simulink model "pfc_closed_loop_ripple4"  (R2016b)
settings: Solver=VariableStepAuto  StartTime=0.0  StopTime=1  RelTol=1e-3
libraries: powerlib x27, simulink x5, powerlib_meascontrol x4
settings Model: SimulationMode=accelerator  Creator=exam  LastModifiedBy=Saagar
settings SolverCC: ZeroCrossAlgorithm=Adaptive

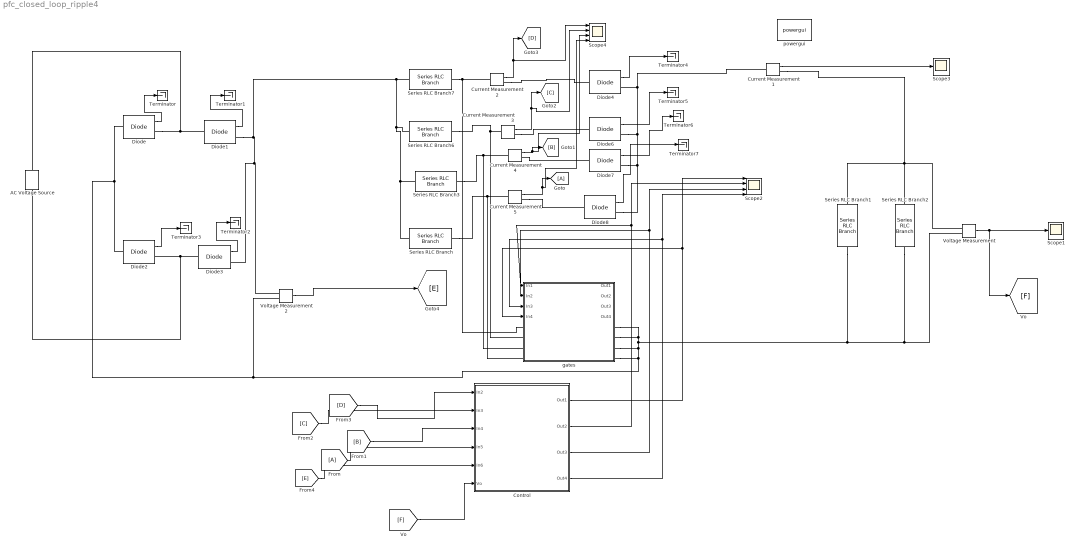
== system pfc_closed_loop_ripple4 ==
  AC Voltage Source : powerlib/Electrical Sources/AC Voltage Source  Amplitude=325  Phase=0  Frequency=50  SampleTime=0  Measurements=None  BusType=swing  Pref=10e3  Qref=0  Qmin=-inf  Qmax=+inf
  Control : Subsystem
  Current Measurement{1..5} (5 alike) : powerlib/Measurements/Current Measurement  PhasorSimulation=off  OutputType=Complex  PSBequivalent=0
  Diode{,1,3..4,6..8} (7 alike) : powerlib/Power Electronics/Diode  Ron=0.001  Lon=0  Vf=0.8  IC=0  UseSnubber=off  Rs=500  Cs=250e-9  Measurements=on
  Diode2 : powerlib/Power Electronics/Diode  Ron=0.001  Lon=0  Vf=0.6  IC=0  UseSnubber=off  Rs=500  Cs=250e-9  Measurements=on
  Scope1 : Scope
  Scope2 : Scope  NumInputPorts=4
  Scope3 : Scope
  Scope4 : Scope  NumInputPorts=4
  Series RLC Branch{,3,6..7} (4 alike) : powerlib/Elements/Series RLC Branch  LConnTagsString=__new0  RConnTagsString=__new0  BranchType=L  Resistance=0  Inductance=0.152e-03  SetiL0=off  InitialCurrent=0  Capacitance=0  Setx0=off  InitialVoltage=0  Measurements=None
  Series RLC Branch1 : powerlib/Elements/Series RLC Branch  LConnTagsString=__new0  RConnTagsString=__new0  BranchType=C  Resistance=0  Inductance=0  SetiL0=off  InitialCurrent=0  Capacitance=4700e-06  Setx0=off  InitialVoltage=0  Measurements=None
  Series RLC Branch2 : powerlib/Elements/Series RLC Branch  LConnTagsString=__new0  RConnTagsString=__new0  BranchType=R  Resistance=150  Inductance=0  SetiL0=off  InitialCurrent=0  Capacitance=10  Setx0=off  InitialVoltage=0  Measurements=None
  Terminator{,1..7} (8 alike) : Terminator
  Voltage Measurement : powerlib/Measurements/Voltage Measurement  PhasorSimulation=off  OutputType=Complex  PSBequivalent=0
  Voltage Measurement2 : powerlib/Measurements/Voltage Measurement  PhasorSimulation=off  OutputType=Complex  PSBequivalent=0
  gates : Subsystem
  powergui : powerlib/powergui  Priority=1  SimulationMode=Continuous  SolverType=Tustin/Backward Euler (TBE)  SampleTime=50e-6  frequency=60  SPID=off  DisableSnubberDevices=off  DisableRonSwitches=off  DisableVfSwitches=off  SwTol=0  DisplayEquations=off  Interpol=off  ExternalGateDelay=off  methode=off  Ts=10  FunctionMessages=off  echomessages=off  HookPort=off  EnableUseOfTLC=off  x0status=blocks  frequencyindice=0  Pbase=100e6  ErrMax=1e-4  Iterations=50  UnitsV=kV  UnitsW=MW  buscounter=0  RestoreLinks=warning  ResistiveCurrentMeasurement=off  Frange=[0:2:500]  Ylog=off  Xlog=on  ShowGrid=off  save=off  variable=ZData  structure=0  ZoomFFT=off  StartTime=0.0  cycles=1  DisplayStyle=1  fundamental=60  FreqAxis=off  MaxFrequency=1000  frequencyindicesteady=1  RmsSteady=1  display=off
  wires:
  Current Measurement1/1 -> Scope3/1
  Voltage Measurement/1 -> Scope1/1, [F]
  Current Measurement2/1 -> Scope4/1, [D]
  Current Measurement5/1 -> Scope4/4, [A]
  Current Measurement4/1 -> Scope4/3, [B]
  Current Measurement3/1 -> Scope4/2, [C]
  Control/4(Out4) -> Scope2/4, gates/3(In3)
  Control/1(Out1) -> Scope2/1, gates/4(In4)
  Control/2(Out2) -> gates/1(In1), Scope2/2
  Control/3(Out3) -> gates/2(In2), Scope2/3
  [D] -> Control/1(In2)
  [C] -> Control/2(In3)
  [B] -> Control/3(In4)
  [A] -> Control/4(In5)
  [E] -> Control/5(In6)
  [F] -> Control/6(Vo)
  Diode/1 -> Terminator/1
  Diode1/1 -> Terminator1/1
  Diode2/1 -> Terminator3/1
  Diode3/1 -> Terminator2/1
  Diode4/1 -> Terminator4/1
  Diode6/1 -> Terminator5/1
  Diode7/1 -> Terminator6/1
  Diode8/1 -> Terminator7/1
  Voltage Measurement2/1 -> [E]
  connections:
  Voltage Measurement/LConn1 -- Series RLC Branch1/LConn1 -- Current Measurement1/RConn1 -- Series RLC Branch2/LConn1
  Diode/RConn1 -- AC Voltage Source/RConn1 -- Diode1/LConn1
  Diode2/RConn1 -- AC Voltage Source/LConn1 -- Diode3/LConn1
  Voltage Measurement/LConn2 -- Series RLC Branch2/RConn1 -- Series RLC Branch1/RConn1 -- Diode2/LConn1 -- Diode/LConn1 -- Voltage Measurement2/LConn2 -- gates/RConn4 -- gates/RConn3 -- gates/RConn1 -- gates/RConn2
  Series RLC Branch7/RConn1 -- gates/LConn1 -- Current Measurement2/LConn1
  Diode7/RConn1 -- Current Measurement1/LConn1 -- Diode4/RConn1 -- Diode6/RConn1 -- Diode8/RConn1
  Current Measurement3/RConn1 -- Diode6/LConn1
  Current Measurement4/RConn1 -- Diode7/LConn1
  Current Measurement5/RConn1 -- Diode8/LConn1
  Series RLC Branch6/RConn1 -- Current Measurement3/LConn1 -- gates/LConn2
  Current Measurement5/LConn1 -- Series RLC Branch/RConn1 -- gates/LConn4
  Series RLC Branch3/RConn1 -- Current Measurement4/LConn1 -- gates/LConn3
  Current Measurement2/RConn1 -- Diode4/LConn1
  Diode1/RConn1 -- Series RLC Branch6/LConn1 -- Series RLC Branch/LConn1 -- Series RLC Branch3/LConn1 -- Series RLC Branch7/LConn1 -- Diode3/RConn1 -- Voltage Measurement2/LConn1

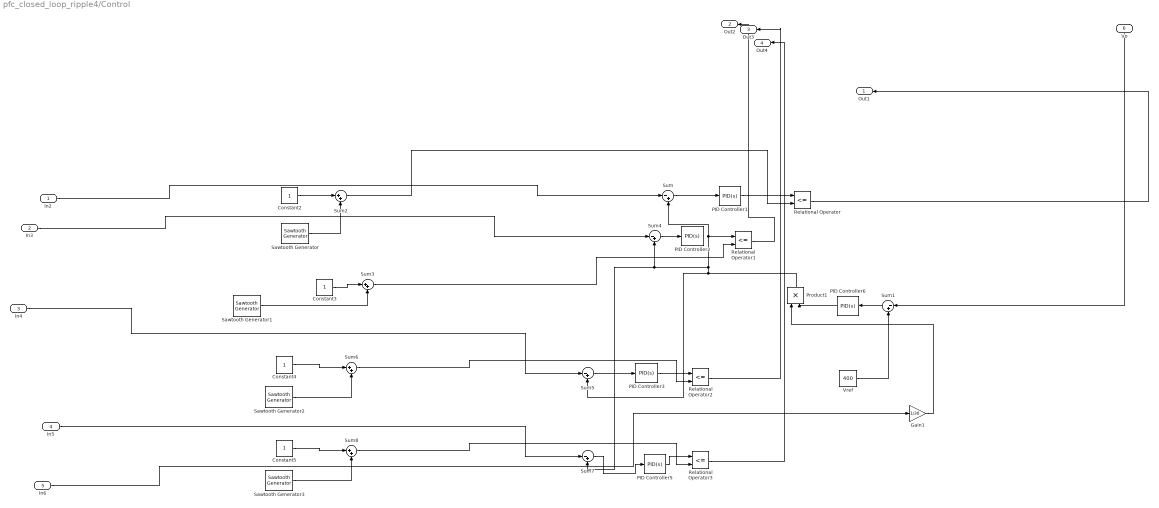
== system pfc_closed_loop_ripple4/Control ==
  In2 : Inport
  In3 : Inport  Port=2
  In4 : Inport  Port=3
  In5 : Inport  Port=4
  In6 : Inport  Port=5
  Vo : Inport  Port=6
  Constant{2..5} (4 alike) : Constant
  Gain1 : Gain  Gain=1/30
  PID Controller{1..3,5..6} (5 alike) : simulink/Continuous/PID Controller  Controller=PID  TimeDomain=Continuous-time  SampleTime=-1  IntegratorMethod=Forward Euler  FilterMethod=Forward Euler  Form=Parallel  UseFilter=on  ControllerParametersSource=internal  P=10  I=10  D=2.5  N=100  InitialConditionSource=internal  InitialConditionForIntegrator=0  InitialConditionForFilter=0  ExternalReset=none  LimitOutput=off  UpperSaturationLimit=inf  LowerSaturationLimit=-inf  LinearizeAsGain=on  AntiWindupMode=none  Kb=1  TrackingMode=off  Kt=1  PParamMin=[]  PParamMax=[]  IParamMin=[]  IParamMax=[]  DParamMin=[]  DParamMax=[]  NParamMin=[]  NParamMax=[]  KbParamMin=[]  KbParamMax=[]  KtParamMin=[]  KtParamMax=[]  POutMin=[]  POutMax=[]  IOutMin=[]  IOutMax=[]  DOutMin=[]  DOutMax=[]  NOutMin=[]  NOutMax=[]  KbOutMin=[]  KbOutMax=[]  KtOutMin=[]  KtOutMax=[]  IntegratorOutMin=[]  IntegratorOutMax=[]  FilterOutMin=[]  FilterOutMax=[]  SumOutMin=[]  SumOutMax=[]  SumI1OutMin=[]  SumI1OutMax=[]  SumI2OutMin=[]  SumI2OutMax=[]  SumI3OutMin=[]  SumI3OutMax=[]  SumDOutMin=[]  SumDOutMax=[]  SaturationOutMin=[]  SaturationOutMax=[]  IntegratorContinuousStateAttributes=''  IntegratorStateMustResolveToSignalObject=off  IntegratorRTWStateStorageClass=Auto  FilterContinuousStateAttributes=''  FilterStateMustResolveToSignalObject=off  FilterRTWStateStorageClass=Auto  DifferentiatorICPrevScaledInput=0  DifferentiatorOutMin=[]  DifferentiatorOutMax=[]
  Product1 : Product
  Relational Operator{,1..3} (4 alike) : RelationalOperator  Operator=<=  OutDataTypeStr=boolean  RndMeth=Simplest
  Sawtooth Generator : powerlib_meascontrol/Pulse & Signal Generators/Sawtooth Generator  Freq=40000  Phase=0  Ts=0
  Sawtooth Generator1 : powerlib_meascontrol/Pulse & Signal Generators/Sawtooth Generator  Freq=40000  Phase=90  Ts=0
  Sawtooth Generator2 : powerlib_meascontrol/Pulse & Signal Generators/Sawtooth Generator  Freq=40000  Phase=180  Ts=0
  Sawtooth Generator3 : powerlib_meascontrol/Pulse & Signal Generators/Sawtooth Generator  Freq=40000  Phase=270  Ts=0
  Sum{,1,4..5,7} (5 alike) : Sum  Inputs=|-+
  Sum{2..3,6,8} (4 alike) : Sum  Inputs=|++
  Vref : Constant  Value=400
  Out1 : Outport
  Out2 : Outport  Port=2
  Out3 : Outport  Port=3
  Out4 : Outport  Port=4
  wires:
  PID Controller6/1 -> Product1/2
  Sum/1 -> PID Controller1/1
  Sawtooth Generator/1 -> Sum2/2
  Constant3/1 -> Sum3/1
  Sawtooth Generator1/1 -> Sum3/2
  Sum3/1 -> Relational Operator1/2
  Constant2/1 -> Sum2/1
  Gain1/1 -> Product1/1
  Sum2/1 -> Relational Operator/2
  PID Controller1/1 -> Relational Operator/1
  Relational Operator/1 -> Out1/1
  Sum1/1 -> PID Controller6/1
  Sum5/1 -> PID Controller3/1
  Relational Operator3/1 -> Out4/1
  Sum8/1 -> Relational Operator3/2
  Relational Operator1/1 -> Out2/1
  Constant5/1 -> Sum8/1
  PID Controller5/1 -> Relational Operator3/1
  Relational Operator2/1 -> Out3/1
  Sum4/1 -> PID Controller2/1
  Sawtooth Generator2/1 -> Sum6/2
  Sum6/1 -> Relational Operator2/2
  PID Controller3/1 -> Relational Operator2/1
  Constant4/1 -> Sum6/1
  Product1/1 -> Sum5/2, Sum7/2, Sum4/2, Relational Operator1/1, Sum/2
  Sum7/1 -> PID Controller5/1
  Sawtooth Generator3/1 -> Sum8/2
  Vo/1 -> Sum1/1
  In5/1 -> Sum7/1
  In6/1 -> Gain1/1
  In2/1 -> Sum/1
  In4/1 -> Sum5/1
  In3/1 -> Sum4/1
  Vref/1 -> Sum1/2

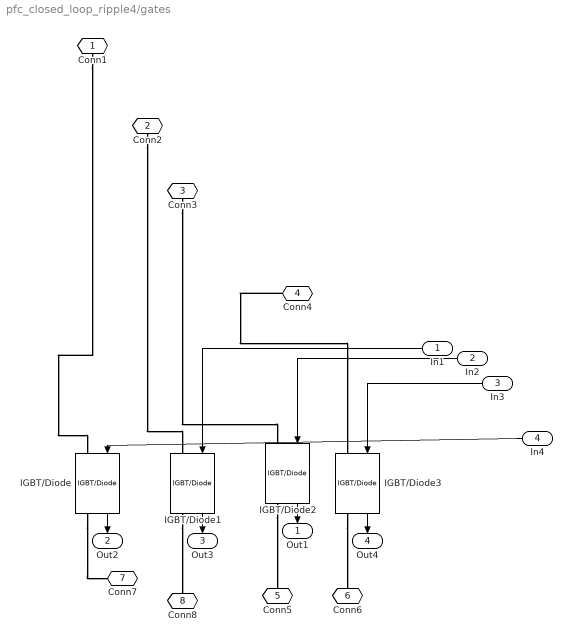
== system pfc_closed_loop_ripple4/gates ==
  In1 : Inport
  In2 : Inport  Port=2
  In3 : Inport  Port=3
  In4 : Inport  Port=4
  IGBT/Diode{,1..3} (4 alike) : powerlib/Power Electronics/IGBT//Diode  Ron=1e-3  Rs=1e5  Cs=inf  Measurements=on
  Conn1 : PMIOPort  Port=1  Side=Left
  Conn2 : PMIOPort  Port=2  Side=Left
  Conn3 : PMIOPort  Port=3  Side=Left
  Conn4 : PMIOPort  Port=4  Side=Left
  Conn5 : PMIOPort  Port=5  Side=Right
  Conn6 : PMIOPort  Port=6  Side=Right
  Conn7 : PMIOPort  Port=7  Side=Right
  Conn8 : PMIOPort  Port=8  Side=Right
  Out1 : Outport
  Out2 : Outport  Port=2
  Out3 : Outport  Port=3
  Out4 : Outport  Port=4
  wires:
  IGBT/Diode/1 -> Out2/1
  IGBT/Diode1/1 -> Out3/1
  IGBT/Diode2/1 -> Out1/1
  In3/1 -> IGBT/Diode3/1
  In1/1 -> IGBT/Diode1/1
  In2/1 -> IGBT/Diode2/1
  IGBT/Diode3/1 -> Out4/1
  In4/1 -> IGBT/Diode/1
  connections:
  IGBT/Diode3/RConn1 -- Conn6/RConn1
  IGBT/Diode2/RConn1 -- Conn5/RConn1
  IGBT/Diode/RConn1 -- Conn7/RConn1
  Conn1/RConn1 -- IGBT/Diode/LConn1
  IGBT/Diode1/RConn1 -- Conn8/RConn1
  Conn3/RConn1 -- IGBT/Diode2/LConn1
  Conn4/RConn1 -- IGBT/Diode3/LConn1
  Conn2/RConn1 -- IGBT/Diode1/LConn1
